simulink model "v40"  (R2014a)
settings: Solver=ode45  StartTime=0.0  StopTime=40360  RelTol=1e-3
libraries: simulink x4
settings Model: NumberOfSteps=15  Creator=zarac  LastModifiedBy=tomii
settings DataIOCC: ReturnWorkspaceOutputs=on
settings SimEventsCC: propDiagAttribOutput=0  propDiagStatOutput=0

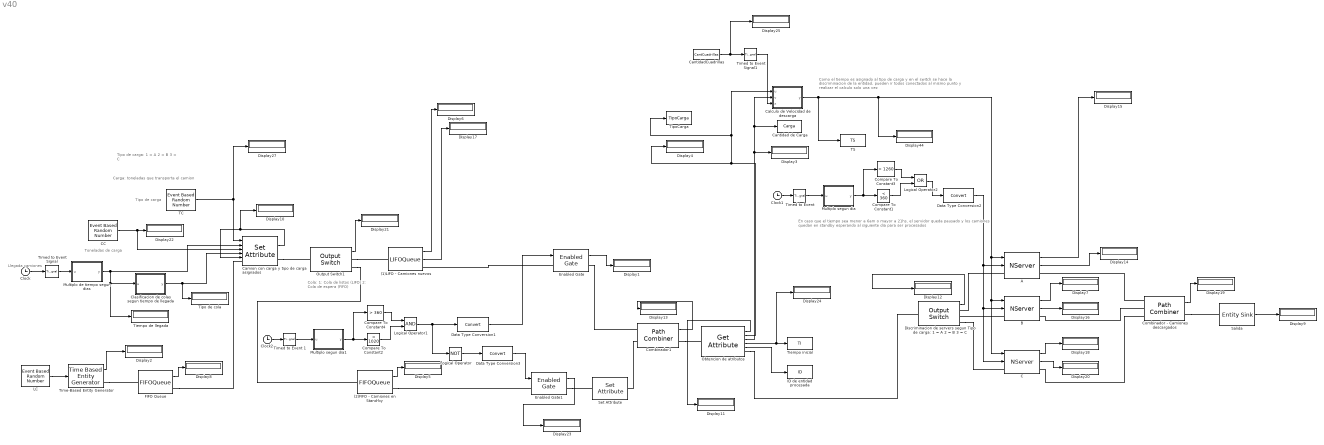
== system v40 ==
  note: Como el tiempo es asignado al tipo de carga y en el switch se hace
      | la discriminacion  de la entidad, pueden ir todos conectados  al mismo
      |  punto y realizar el calculo solo una vez
  note: En caso que el tiempo sea menor a 6am o mayor a 21hs, el servidor queda pausado y los
      | camiones quedan en standby esperando al siguiente dia para ser procesados
  note: Tipo de carga:
      | 1 = A
      | 2 = B
      | 3 = C
  note: Llegada camiones
  note: Toneladas de carga
  note: Tipo de carga
  note: Carga: toneladas que transporta el camion
  note: Cola:
      | 1: Cola de listos (LIFO)
      | 2: Cola de espera (FIFO)
  (1)LIFO - Camiones nuevos : LIFOQueue  Capacity=inf  StatNumberDeparted=on  StatNumberInBlock=on
      settings: OutputPortMap=o0,o1
  (2)FIFO - Camiones en Stand-by : FIFOQueue  Capacity=inf  StatNumberDeparted=on
  A : NServer  NumberOfServers=1  ServiceTimeFrom=Signal port t  AllowServiceControl=on  StatNumberDeparted=on  StatNumberInBlock=on
      settings: InputPortMap=u0,u1  OutputPortMap=o0,o1
  B : NServer  NumberOfServers=1  ServiceTimeFrom=Signal port t  AllowServiceControl=on  StatNumberDeparted=on  StatNumberInBlock=on
      settings: InputPortMap=u0,u1  OutputPortMap=o0,o1
  C : NServer  NumberOfServers=1  ServiceTimeFrom=Signal port t  AllowServiceControl=on  StatNumberDeparted=on  StatNumberInBlock=on
      settings: InputPortMap=u0,u1  OutputPortMap=o0,o1
  CC : EventBasedRandomNumber  Distribution=Gaussian (normal)  meanNorm=20  stdNorm=3.5  Seed=462317
  Calculo de Velocidad de descarga : MATLAB Function  TreatAsAtomicUnit=on
  Camion con carga y tipo de carga asignados : SetAttribute  AttributeName=TipoDeCarga|Tiempo|PrecioBase|Carga|Desicion|Cola|ID  AttributeFrom=Signal port|Signal port|Dialog|Signal port|Dialog|Signal port|Signal port  AttributeValue=1|clock|94|1|1|1|1  AttributeTreatAsVector=1|1|1|1|1|1|1  StatNumberDeparted=on  EvaluatedAttributeValue={ [];[];94;[];1;[];[]}
      settings: InputPortMap=u0,u1,u3,u5,u6
  Cantidad de Carga : ToWorkspace  VariableName=Carga  SaveFormat=Timeseries  SampleTime=-1
  CantidadCuadrillas : FromWorkspace  VariableName=CantCuadrillas  SampleTime=0
  Clasificacion de colas segun tiempo de llegada : MATLAB Function  TreatAsAtomicUnit=on
  Clock : Clock
  Clock1 : Clock
  Clock2 : Clock
  Combinador - Camiones descargados : PathCombiner  StatNumberDeparted=on
  Combinador1 : PathCombiner  NumberInputPorts=2  StatNumberDeparted=on
  Compare To Constant1 : simulink/Logic and Bit Operations/Compare To Constant  relop=<  const=360  OutDataTypeStr=uint8
  Compare To Constant2 : simulink/Logic and Bit Operations/Compare To Constant  relop=<  const=1020  OutDataTypeStr=uint8
  Compare To Constant3 : simulink/Logic and Bit Operations/Compare To Constant  relop=>  const=1260  OutDataTypeStr=uint8
  Compare To Constant4 : simulink/Logic and Bit Operations/Compare To Constant  relop=>  const=360  OutDataTypeStr=uint8
  Data Type Conversion1 : DataTypeConversion  OutMin=[-1]  OutMax=[1]
  Data Type Conversion2 : DataTypeConversion  OutMin=[-1]  OutMax=[1]
  Data Type Conversion3 : DataTypeConversion  OutMin=[-1]  OutMax=[1]
  "Discriminacion de servers segun Tipo de carga: 1 = A 2 = B 3 = C " : OutputSwitch  StatNumberDeparted=on
  Display{1..25,27,44} (27 alike) : Display
      Display19 settings: Decimation=2
  Enabled Gate : EnabledGate  StatNumberDeparted=on
  Enabled Gate1 : EnabledGate  StatNumberDeparted=on
  FIFO Queue : FIFOQueue  Capacity=inf  StatNumberInBlock=on
      settings: OutputPortMap=o1
  ID de entidad procesada : ToWorkspace  VariableName=ID  SaveFormat=Timeseries  SampleTime=-1
  LC : EventBasedRandomNumber  meanExp=2.466  meanNorm=20  stdNorm=3.5  Seed=150794
  Logical Operator : Logic  Operator=NOT  AllPortsSameDT=off  OutDataTypeStr=boolean
  Logical Operator1 : Logic  AllPortsSameDT=off  OutDataTypeStr=boolean
  Logical Operator2 : Logic  Operator=OR  AllPortsSameDT=off  OutDataTypeStr=boolean
  Multiplo de tiempo segun dias : MATLAB Function  TreatAsAtomicUnit=on
  Multiplo segun dia : MATLAB Function  TreatAsAtomicUnit=on
  Multiplo segun dia1 : MATLAB Function  TreatAsAtomicUnit=on
  Obtencion de atributos : GetAttribute  AttributeName=TipoDeCarga|Carga|Tiempo|ID  AttributeMissing=Error|Error|Error|Error  AttributeDefaultValue=1|1|1|1  AttributeTreatAsVector=1|1|1|1  AttributeSendTiming=After entity departure|After entity departure|After entity departure|After entity departure  StatNumberDeparted=on  EvaluatedDefaultAttributeValue={ [];[];[];[]}
      settings: OutputPortMap=o0,o1,o2,o3,o4
  Output Switch1 : OutputSwitch  NumberOutputPorts=2  SwitchingCriterion=From attribute  AttributeName=Cola  StatNumberDeparted=on
  "Salida " : EntitySink  StatNumberArrived=on
  Set Attribute : SetAttribute  AttributeName=Tiempo  AttributeValue=360  EvaluatedAttributeValue={ 360}
  TC : EventBasedRandomNumber  Distribution=Arbitrary discrete  valueVecDisc=[1 2 3]  probVecDisc=[0.4 0.35 0.25]  Seed=425890
  TS : ToWorkspace  VariableName=TS  SaveFormat=Timeseries  SampleTime=-1
  Tiempo de llegada : Display
  Tiempo inicial : ToWorkspace  VariableName=TI  SaveFormat=Timeseries  SampleTime=-1
  Time-Based Entity Generator : TimeBasedEntityGenerator  GenerateEntitiesUpon=Intergeneration time from port t  Distribution=Exponential  InitialSeed=567498  Mean=2.46  StatNumberDeparted=on
  "Timed to Event " : TimedToEventSignal
  Timed to Event 1 : TimedToEventSignal
  Timed to Event Signal : TimedToEventSignal
  Timed to Event Signal1 : TimedToEventSignal
  Tipo de cola : Display
  TipoCarga : ToWorkspace  VariableName=TipoCarga  SaveFormat=Timeseries  SampleTime=-1
  wires:
  (1)LIFO - Camiones nuevos/1 -> Display6/1
  LC/1 -> Time-Based Entity Generator/1
  Clock/1 -> Timed to Event Signal/1
  B/1 -> Display7/1
  "Salida "/1 -> Display9/1
  (1)LIFO - Camiones nuevos/2 -> Display17/1
  CC/1 -> Display22/1, Camion con carga y tipo de carga asignados/3
  TC/1 -> Camion con carga y tipo de carga asignados/1, Display27/1
  Time-Based Entity Generator/1 -> Display2/1
  Camion con carga y tipo de carga asignados/1 -> Camion con carga y tipo de carga asignados/5, Display10/1
  Timed to Event Signal/1 -> Multiplo de tiempo segun dias/1(u)
  Clasificacion de colas segun tiempo de llegada/1(y) -> Camion con carga y tipo de carga asignados/4, Tipo de cola/1
  Calculo de Velocidad de descarga/1(y) -> TS/1, A/1, B/1, C/1, Display44/1
  Obtencion de atributos/2 -> Display4/1, TipoCarga/1, Calculo de Velocidad de descarga/1(u)
  Obtencion de atributos/3 -> Display3/1, Cantidad de Carga/1, Calculo de Velocidad de descarga/2(v)
  Multiplo de tiempo segun dias/1(y) -> Tiempo de llegada/1, Clasificacion de colas segun tiempo de llegada/1(u), Camion con carga y tipo de carga asignados/2
  "Discriminacion de servers segun Tipo de carga: 1 = A 2 = B 3 = C "/1 -> Display12/1
  A/1 -> Display15/1
  C/1 -> Display18/1
  Combinador - Camiones descargados/1 -> Display19/1
  Clock1/1 -> "Timed to Event "/1
  Compare To Constant3/1 -> Logical Operator2/1
  Compare To Constant1/1 -> Logical Operator2/2
  Logical Operator2/1 -> Data Type Conversion2/1
  "Timed to Event "/1 -> Multiplo segun dia/1(u)
  Multiplo segun dia/1(y) -> Compare To Constant1/1, Compare To Constant3/1
  Data Type Conversion2/1 -> A/2, B/2, C/2
  Clock2/1 -> Timed to Event 1/1
  Compare To Constant4/1 -> Logical Operator1/1
  Compare To Constant2/1 -> Logical Operator1/2
  Logical Operator1/1 -> Logical Operator/1, Data Type Conversion1/1
  Timed to Event 1/1 -> Multiplo segun dia1/1(u)
  Multiplo segun dia1/1(y) -> Compare To Constant2/1, Compare To Constant4/1
  Data Type Conversion1/1 -> Enabled Gate/1
  Enabled Gate/1 -> Display1/1
  FIFO Queue/1 -> Display8/1
  Logical Operator/1 -> Data Type Conversion3/1
  (2)FIFO - Camiones en Stand-by/1 -> Display5/1
  Combinador1/1 -> Display13/1
  Data Type Conversion3/1 -> Enabled Gate1/1
  A/2 -> Display14/1
  B/2 -> Display16/1
  C/2 -> Display20/1
  Output Switch1/1 -> Display21/1
  Enabled Gate1/1 -> Display23/1
  Obtencion de atributos/1 -> Display11/1
  Obtencion de atributos/4 -> Display24/1, Tiempo inicial/1
  Obtencion de atributos/5 -> ID de entidad procesada/1
  CantidadCuadrillas/1 -> Display25/1, Timed to Event Signal1/1
  Timed to Event Signal1/1 -> Calculo de Velocidad de descarga/3(x)
  connections:
  Combinador - Camiones descargados/RConn1 -- "Salida "/LConn1
  A/LConn1 -- "Discriminacion de servers segun Tipo de carga: 1 = A 2 = B 3 = C "/RConn1
  B/LConn1 -- "Discriminacion de servers segun Tipo de carga: 1 = A 2 = B 3 = C "/RConn2
  "Discriminacion de servers segun Tipo de carga: 1 = A 2 = B 3 = C "/RConn3 -- C/LConn1
  Combinador - Camiones descargados/LConn1 -- A/RConn1
  Combinador - Camiones descargados/LConn2 -- B/RConn1
  Combinador - Camiones descargados/LConn3 -- C/RConn1
  Enabled Gate/LConn1 -- (1)LIFO - Camiones nuevos/RConn1
  FIFO Queue/RConn1 -- Camion con carga y tipo de carga asignados/LConn1
  Time-Based Entity Generator/RConn1 -- FIFO Queue/LConn1
  (2)FIFO - Camiones en Stand-by/RConn1 -- Enabled Gate1/LConn1
  Combinador1/RConn1 -- Obtencion de atributos/LConn1
  Enabled Gate/RConn1 -- Combinador1/LConn1
  Set Attribute/RConn1 -- Combinador1/LConn2
  Camion con carga y tipo de carga asignados/RConn1 -- Output Switch1/LConn1
  Output Switch1/RConn1 -- (1)LIFO - Camiones nuevos/LConn1
  Output Switch1/RConn2 -- (2)FIFO - Camiones en Stand-by/LConn1
  Obtencion de atributos/RConn1 -- "Discriminacion de servers segun Tipo de carga: 1 = A 2 = B 3 = C "/LConn1
  Enabled Gate1/RConn1 -- Set Attribute/LConn1

== matlab function v40/Calculo de Velocidad de descarga ==
  data: u input; y output; v input; x input
function y = fcn(u, v, x)
    % x: cantidad de cuadrillas
    % u: tipo de carga
    % v: cantidad de carga

if u == 1
    velocidad = x * (6 / 60); % Tipo de carga 1
elseif u == 2
    velocidad = x * (5.5 / 60); % Tipo de carga 2
elseif u == 3
    velocidad = x * (3.5 / 60); % Tipo de carga 3
else
    v = 0;
    velocidad = 1;
end


    % Calcular el tiempo necesario para descargar la carga
    y = v / velocidad;
end

== matlab function v40/Multiplo de tiempo segun dias ==
  data: u input; y output
function y= fcn(u)
    %u es el valor de tiempo en minutos
    y = mod(u, 1440); 
 end

== matlab function v40/Multiplo segun dia1 ==
  data: u input; y output
function y= fcn(u)
    %u es el valor de tiempo en minutos
    y = mod(u, 1440); 
 end

== matlab function v40/Clasificacion de colas segun tiempo de llegada ==
  data: u input; y output
function y = fcn(u)
    %u es el valor de tiempo en minutos
    %1 es cola de listos
    %2 es cola de espera
    minutos = u;

    if minutos >= 360 && minutos <= 1020  %Si llegan entre 6am y 17pm, van a cola de listos
         cola = 1;
         %fprintf('Cola: %.2f , Horario: %.2f\n', cola,minutos); %Imprimo por pantalla para ver si est todo bien
        
    else 
        cola = 2; %En caso contrario, van a cola espera
         %fprintf('Cola: %.2f , Horario: %.2f\n', cola,minutos); %Imprimo por pantalla para ver si est todo bien
    end 
    y = cola;
end

== matlab function v40/Multiplo segun dia ==
  data: u input; y output
function y= fcn(u)
    %u es el valor de tiempo en minutos
    y = mod(u, 1440); 
 end
